simulink model "SF051A_SnsrOffsLrng"  (R2013b)
settings: Solver=FixedStepDiscrete  SolverMode=SingleTasking  StartTime=0.0  StopTime=1  FixedStep=0.002  RelTol=1e-3
values from neighbouring files (symbols this model uses):
  ARCHGLBPRM_10MILLISEC_SEC_F32 = DataDict.Constant    [SF051A_SnsrOffsLrng_DataDict.m]
  ARCHGLBPRM_2MILLISEC_SEC_F32 = DataDict.Constant    [SF051A_SnsrOffsLrng_DataDict.m]
  ARCHGLBPRM_2PI_ULS_F32 = DataDict.Constant    [SF051A_SnsrOffsLrng_DataDict.m]
  ARCHGLBPRM_FLOATZEROTHD_ULS_F32 = DataDict.Constant    [SF051A_SnsrOffsLrng_DataDict.m]
  ARCHGLBPRM_PIOVER180_ULS_F32 = DataDict.Constant    [SF051A_SnsrOffsLrng_DataDict.m]
  CNV100MICROSECTOSEC_SECPERCNT_F32 = DataDict.Constant    [SF051A_SnsrOffsLrng_DataDict.m]
  COVRAMTRXNIT_ULS_F32 = DataDict.Constant    [SF051A_SnsrOffsLrng_DataDict.m]
  HWAGHILIM_HWDEG_F32 = DataDict.Constant    [SF051A_SnsrOffsLrng_DataDict.m]
  HWAUTHYTHD_ULS_F32 = DataDict.Constant    [SF051A_SnsrOffsLrng_DataDict.m]
  HWTQLRNGSTSLRND_CNT_U08 = DataDict.Constant    [SF051A_SnsrOffsLrng_DataDict.m]
  HWTQLRNGSTSNEGOFFS_CNT_U08 = DataDict.Constant    [SF051A_SnsrOffsLrng_DataDict.m]
  HWTQLRNGSTSNOTLRND_CNT_U08 = DataDict.Constant    [SF051A_SnsrOffsLrng_DataDict.m]
  HWTQLRNGSTSPOSOFFS_CNT_U08 = DataDict.Constant    [SF051A_SnsrOffsLrng_DataDict.m]
  HWTQLRNGSTSZEROOFFS_CNT_U08 = DataDict.Constant    [SF051A_SnsrOffsLrng_DataDict.m]
  IDYMTRX_ULS_F32 = DataDict.Constant    [SF051A_SnsrOffsLrng_DataDict.m]
  IVS10MS_ULSPERSEC_F32 = DataDict.Constant    [SF051A_SnsrOffsLrng_DataDict.m]
  LRNGFILTICON_ULS_F32 = DataDict.Constant    [SF051A_SnsrOffsLrng_DataDict.m]
  ONE_ULS_F32 = DataDict.Constant    [SF051A_SnsrOffsLrng_DataDict.m]
  SnsrOffsLrnd = DataDict.NVM    [SF051A_SnsrOffsLrng_DataDict.m]
  SnsrOffsLrngFctEna = DataDict.Calibration    [SF051A_SnsrOffsLrng_DataDict.m]
  SnsrOffsLrngHwAgLrngDrvgDstThd = DataDict.Calibration    [SF051A_SnsrOffsLrng_DataDict.m]
  SnsrOffsLrngHwAgLrngEna = DataDict.Calibration    [SF051A_SnsrOffsLrng_DataDict.m]
  SnsrOffsLrngHwAgLrngHwVelThd = DataDict.Calibration    [SF051A_SnsrOffsLrng_DataDict.m]
  SnsrOffsLrngHwAgLrngSysTqThd = DataDict.Calibration    [SF051A_SnsrOffsLrng_DataDict.m]
  SnsrOffsLrngHwAgLrngSysTqThdMed = DataDict.Calibration    [SF051A_SnsrOffsLrng_DataDict.m]
  SnsrOffsLrngHwAgLrngSysTqThdTrustd = DataDict.Calibration    [SF051A_SnsrOffsLrng_DataDict.m]
  SnsrOffsLrngHwAgLrngSysTqThdWide = DataDict.Calibration    [SF051A_SnsrOffsLrng_DataDict.m]
  SnsrOffsLrngHwAgLrngTi = DataDict.Calibration    [SF051A_SnsrOffsLrng_DataDict.m]
  SnsrOffsLrngHwAgLrngVehSpdThd = DataDict.Calibration    [SF051A_SnsrOffsLrng_DataDict.m]
  SnsrOffsLrngHwAgLrngYawOffsDbnd = DataDict.Calibration    [SF051A_SnsrOffsLrng_DataDict.m]
  SnsrOffsLrngHwAgLrngYawRateThd = DataDict.Calibration    [SF051A_SnsrOffsLrng_DataDict.m]
  SnsrOffsLrngHwAgOffsLim = DataDict.Calibration    [SF051A_SnsrOffsLrng_DataDict.m]
  SnsrOffsLrngHwTqLrngEna = DataDict.Calibration    [SF051A_SnsrOffsLrng_DataDict.m]
  SnsrOffsLrngHwTqLrngEnaTiThd = DataDict.Calibration    [SF051A_SnsrOffsLrng_DataDict.m]
  SnsrOffsLrngHwTqLrngHwAgDbnd = DataDict.Calibration    [SF051A_SnsrOffsLrng_DataDict.m]
  SnsrOffsLrngHwTqLrngHwAgThd = DataDict.Calibration    [SF051A_SnsrOffsLrng_DataDict.m]
  SnsrOffsLrngHwTqLrngHwTqThd = DataDict.Calibration    [SF051A_SnsrOffsLrng_DataDict.m]
  SnsrOffsLrngHwTqLrngHwTqZeroOffsThd = DataDict.Calibration    [SF051A_SnsrOffsLrng_DataDict.m]
  SnsrOffsLrngHwTqLrngHwVelThd = DataDict.Calibration    [SF051A_SnsrOffsLrng_DataDict.m]
  SnsrOffsLrngHwTqLrngMeasTi = DataDict.Calibration    [SF051A_SnsrOffsLrng_DataDict.m]
  SnsrOffsLrngHwTqLrngMeasTiScar = DataDict.Calibration    [SF051A_SnsrOffsLrng_DataDict.m]
  SnsrOffsLrngHwTqLrngSampleImbThd1 = DataDict.Calibration    [SF051A_SnsrOffsLrng_DataDict.m]
  SnsrOffsLrngHwTqLrngSampleImbThd2 = DataDict.Calibration    [SF051A_SnsrOffsLrng_DataDict.m]
  SnsrOffsLrngHwTqLrngSampleThd1 = DataDict.Calibration    [SF051A_SnsrOffsLrng_DataDict.m]
  SnsrOffsLrngHwTqLrngSampleThd2 = DataDict.Calibration    [SF051A_SnsrOffsLrng_DataDict.m]
  SnsrOffsLrngHwTqLrngTiWghtCoeff = DataDict.Calibration    [SF051A_SnsrOffsLrng_DataDict.m]
  SnsrOffsLrngHwTqLrngVehSpdThd = DataDict.Calibration    [SF051A_SnsrOffsLrng_DataDict.m]
  SnsrOffsLrngHwTqOffsLim = DataDict.Calibration    [SF051A_SnsrOffsLrng_DataDict.m]
  SnsrOffsLrngSampleCntForHwTqLrngRst = DataDict.Calibration    [SF051A_SnsrOffsLrng_DataDict.m]
  SnsrOffsLrngTqInpDetnPwrEstimnThd = DataDict.Calibration    [SF051A_SnsrOffsLrng_DataDict.m]
  SnsrOffsLrngTqInpDetnSinGenrAmp = DataDict.Calibration    [SF051A_SnsrOffsLrng_DataDict.m]
  SnsrOffsLrngTqInpDetnSinGenrFrq = DataDict.Calibration    [SF051A_SnsrOffsLrng_DataDict.m]
  SnsrOffsLrngTqInpDetnStg1FilGain = DataDict.Calibration    [SF051A_SnsrOffsLrng_DataDict.m]
  SnsrOffsLrngTqInpDetnStg1WinSize = DataDict.Calibration    [SF051A_SnsrOffsLrng_DataDict.m]
  SnsrOffsLrngTqInpDetnStg2FilGainCen = DataDict.Calibration    [SF051A_SnsrOffsLrng_DataDict.m]
  SnsrOffsLrngTqInpDetnStg2FilGainDwn = DataDict.Calibration    [SF051A_SnsrOffsLrng_DataDict.m]
  SnsrOffsLrngTqInpDetnStg2FilGainUp = DataDict.Calibration    [SF051A_SnsrOffsLrng_DataDict.m]
  SnsrOffsLrngTqInpDetnStg2WinSize = DataDict.Calibration    [SF051A_SnsrOffsLrng_DataDict.m]
  SnsrOffsLrngYawLrngEna = DataDict.Calibration    [SF051A_SnsrOffsLrng_DataDict.m]
  SnsrOffsLrngYawLrngHwAgThd = DataDict.Calibration    [SF051A_SnsrOffsLrng_DataDict.m]
  SnsrOffsLrngYawLrngTi = DataDict.Calibration    [SF051A_SnsrOffsLrng_DataDict.m]
  SnsrOffsLrngYawLrngYawAThd = DataDict.Calibration    [SF051A_SnsrOffsLrng_DataDict.m]
  SnsrOffsLrngYawOffsFrshTiThd = DataDict.Calibration    [SF051A_SnsrOffsLrng_DataDict.m]
  SnsrOffsLrngYawRateOffsLim = DataDict.Calibration    [SF051A_SnsrOffsLrng_DataDict.m]
  SPDCNVN_MTRPERSECPERKPH_F32 = DataDict.Constant    [SF051A_SnsrOffsLrng_DataDict.m]
  SysGlbPrmSysTqRat = DataDict.ImprtdCal    [SF051A_SnsrOffsLrng_DataDict.m]
  TISTEP10MS_MINS_F32 = DataDict.Constant    [SF051A_SnsrOffsLrng_DataDict.m]
  TQINPDETNLOGGAIN_ULS_F32 = DataDict.Constant    [SF051A_SnsrOffsLrng_DataDict.m]
  YAWELPDTIHILIM_MINS_F32 = DataDict.Constant    [SF051A_SnsrOffsLrng_DataDict.m]
  YAWRATENOISE_VEHDEGPERSEC_F32 = DataDict.Constant    [SF051A_SnsrOffsLrng_DataDict.m]
  ZERO_ULS_F32 = DataDict.Constant    [SF051A_SnsrOffsLrng_DataDict.m]
  ZEROVECT_ULS_F32 = DataDict.Constant    [SF051A_SnsrOffsLrng_DataDict.m]
undefined symbols (not defined in the file or in its folder): NvmGetErrSts1
libraries: Fil x34, NxtrLim x20, FixdToFloat x17, FloatToFixd x16, simulink x12, NxtrAbslt x12, NxtrNvM x8, NxtrMath x3
(part 8 of 12)

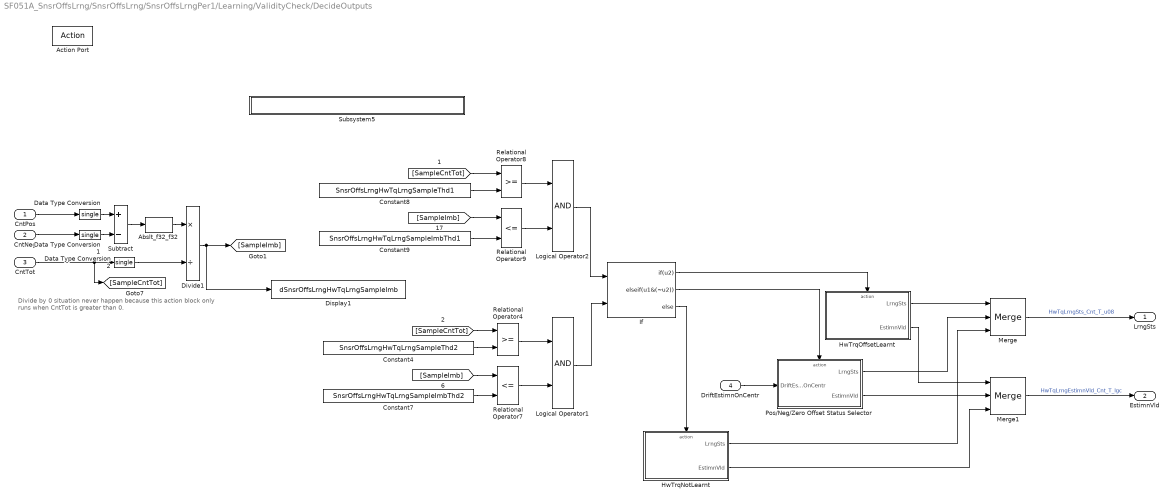
== system SF051A_SnsrOffsLrng/SnsrOffsLrng/SnsrOffsLrngPer1/Learning/ValidityCheck/DecideOutputs ==
  note: Divide by 0 situation never happen because this
      | action block only runs when CntTot is greater than 0.
  CntPos : Inport
  CntNeg : Inport  Port=2
  CntTot : Inport  Port=3
  DriftEstimnOnCentr : Inport  Port=4
  Action Port : ActionPort  ActionType=then
  Abslt_f32_f32 : NxtrAbslt/Abslt_f32_f32  SFunctionSpec=single y1 = Abslt_f32_f32(single u1)
      settings: AttributesFormatString=%<Name>
  Constant4 : Constant  RequirementInfo="{'linktype_rmi_doors' '0000babd (/E-STEER Core/SubSystem Specifications/Application Functions/SF051A Sensor Offset Learning)' '#SF051A_191' 'true' 'REQ:  SF051A_191' '' } %GIDa_69e41f1c_0c44_40e9_b72f_03bb47ca0505"  Value=SnsrOffsLrngHwTqLrngSampleThd2
  Constant7 : Constant  RequirementInfo="{'linktype_rmi_doors' '0000babd (/E-STEER Core/SubSystem Specifications/Application Functions/SF051A Sensor Offset Learning)' '#SF051A_191' 'true' 'REQ:  SF051A_191' '' } %GIDa_92758992_3392_4f8d_bbc2_47c47a841263"  Value=SnsrOffsLrngHwTqLrngSampleImbThd2
  Constant8 : Constant  RequirementInfo="{'linktype_rmi_doors' '0000babd (/E-STEER Core/SubSystem Specifications/Application Functions/SF051A Sensor Offset Learning)' '#SF051A_186' 'true' 'REQ: SF051A_186' '' ; 'linktype_rmi_doors' '0000babd (/E-STEER Core/SubSystem Specifications/Application Functions/SF051A Sensor Offset Learning)' '#SF051A_195' 'true' 'REQ:  SF051A_195' '' ; 'linktype_rmi_doors' '0000babd (/E-STEER Core/SubSystem Specifications/Application Functions/SF051A Sensor Offset Learning)' '#SF051A_194' 'true' 'REQ:  SF051A_194' '' } %GIDa_ce699618_5d0a_4879_9841_5152f833be51"  Value=SnsrOffsLrngHwTqLrngSampleThd1
  Constant9 : Constant  RequirementInfo="{'linktype_rmi_doors' '0000babd (/E-STEER Core/SubSystem Specifications/Application Functions/SF051A Sensor Offset Learning)' '#SF051A_186' 'true' 'REQ: SF051A_186' '' ; 'linktype_rmi_doors' '0000babd (/E-STEER Core/SubSystem Specifications/Application Functions/SF051A Sensor Offset Learning)' '#SF051A_195' 'true' 'REQ:  SF051A_195' '' ; 'linktype_rmi_doors' '0000babd (/E-STEER Core/SubSystem Specifications/Application Functions/SF051A Sensor Offset Learning)' '#SF051A_194' 'true' 'REQ:  SF051A_194' '' } %GIDa_77d3a507_06ae_4bbf_9b68_48e8353a45e0"  Value=SnsrOffsLrngHwTqLrngSampleImbThd1
  Data Type Conversion : DataTypeConversion  OutDataTypeStr=single
  Data Type Conversion1 : DataTypeConversion  OutDataTypeStr=single
  Data Type Conversion2 : DataTypeConversion  OutDataTypeStr=single
  Display1 : DataStoreWrite  DataStoreName=dSnsrOffsLrngHwTqLrngSampleImb
  Divide1 : Product  Inputs=*/
  HwTrqNotLearnt : Subsystem  RequirementInfo="{'linktype_rmi_doors' '0000babd (/E-STEER Core/SubSystem Specifications/Application Functions/SF051A Sensor Offset Learning)' '#SF051A_188' 'true' 'REQ:  SF051A_188' '' } %GIDa_0852b3e3_8f60_4c1b_a1ce_1713cda0b42d"  TreatAsAtomicUnit=on
  HwTrqOffsetLearnt : Subsystem  RequirementInfo="{'linktype_rmi_doors' '0000babd (/E-STEER Core/SubSystem Specifications/Application Functions/SF051A Sensor Offset Learning)' '#SF051A_191' 'true' 'REQ:  SF051A_191' '' ; 'linktype_rmi_doors' '0000babd (/E-STEER Core/SubSystem Specifications/Application Functions/SF051A Sensor Offset Learning)' '#SF051A_187' 'true' 'REQ:  SF051A_187' '' } %GIDa_a502fd14_57b6_42c3_a417_d587305743af"  TreatAsAtomicUnit=on
  If : If  RequirementInfo="{'linktype_rmi_doors' '0000babd (/E-STEER Core/SubSystem Specifications/Application Functions/SF051A Sensor Offset Learning)' '#SF051A_191' 'true' 'REQ: SF051A_191' '' ; 'linktype_rmi_doors' '0000babd (/E-STEER Core/SubSystem Specifications/Application Functions/SF051A Sensor Offset Learning)' '#SF051A_188' 'true' 'REQ:  SF051A_188' '' ; 'linktype_rmi_doors' '0000babd (/E-STEER Core/SubSystem Specifications/Application Functions/SF051A Sensor Offset Learning)' '#SF051A_187' 'true' 'REQ:  SF051A_187' '' ; 'linktype_rmi_doors' '0000babd (/E-STEER Core/SubSystem Specifications/Application Functions/SF051A Sensor Offset Learning)' '#SF051A_186' 'true' 'REQ:  SF051A_186' '' ; 'linktype_rmi_doors' '0000babd (/E-STEER Core/SubSystem Specifications/Application Functions/SF051A Sensor Offset Learning)' '#SF051A_195' 'true' 'REQ:  SF051A_195' '' ; 'linktype_rmi_doors' '0000babd (/E-STEER Core/SubSystem Specifications/Application Functions/SF051A Sensor Offset Learning)' '#SF051A_194' 'true' 'REQ:  SF051A_194' '' } %GIDa_3b80c21c_9329_459d_81b8_15c83f98be44"  NumInputs=2  IfExpression=u2  ElseIfExpressions=u1&(~u2)
  Logical Operator1 : Logic  RequirementInfo="{'linktype_rmi_doors' '0000babd (/E-STEER Core/SubSystem Specifications/Application Functions/SF051A Sensor Offset Learning)' '#SF051A_191' 'true' 'REQ:  SF051A_191' '' } %GIDa_0d8d9f4f_132b_432e_bde6_871d76097d27"  AllPortsSameDT=off  OutDataTypeStr=boolean
  Logical Operator2 : Logic  RequirementInfo="{'linktype_rmi_doors' '0000babd (/E-STEER Core/SubSystem Specifications/Application Functions/SF051A Sensor Offset Learning)' '#SF051A_186' 'true' 'REQ: SF051A_186' '' ; 'linktype_rmi_doors' '0000babd (/E-STEER Core/SubSystem Specifications/Application Functions/SF051A Sensor Offset Learning)' '#SF051A_195' 'true' 'REQ:  SF051A_195' '' ; 'linktype_rmi_doors' '0000babd (/E-STEER Core/SubSystem Specifications/Application Functions/SF051A Sensor Offset Learning)' '#SF051A_194' 'true' 'REQ:  SF051A_194' '' } %GIDa_51f40efb_db01_49b1_90e1_88342bdb2bcc"  AllPortsSameDT=off  OutDataTypeStr=boolean
  Merge : Merge  Inputs=3
  Merge1 : Merge  Inputs=3
  Pos/Neg/Zero Offset Status Selector : Subsystem  TreatAsAtomicUnit=on
  Relational Operator4 : RelationalOperator  RequirementInfo="{'linktype_rmi_doors' '0000babd (/E-STEER Core/SubSystem Specifications/Application Functions/SF051A Sensor Offset Learning)' '#SF051A_191' 'true' 'REQ:  SF051A_191' '' } %GIDa_e4ce5424_fe6e_4165_9ce9_8a105b03caf7"  OutDataTypeStr=boolean
  Relational Operator7 : RelationalOperator  RequirementInfo="{'linktype_rmi_doors' '0000babd (/E-STEER Core/SubSystem Specifications/Application Functions/SF051A Sensor Offset Learning)' '#SF051A_191' 'true' 'REQ:  SF051A_191' '' } %GIDa_9020cee8_144c_4ac3_9e5a_358b6b128393"  Operator=<=  OutDataTypeStr=boolean
  Relational Operator8 : RelationalOperator  RequirementInfo="{'linktype_rmi_doors' '0000babd (/E-STEER Core/SubSystem Specifications/Application Functions/SF051A Sensor Offset Learning)' '#SF051A_186' 'true' 'REQ: SF051A_186' '' ; 'linktype_rmi_doors' '0000babd (/E-STEER Core/SubSystem Specifications/Application Functions/SF051A Sensor Offset Learning)' '#SF051A_195' 'true' 'REQ:  SF051A_195' '' ; 'linktype_rmi_doors' '0000babd (/E-STEER Core/SubSystem Specifications/Application Functions/SF051A Sensor Offset Learning)' '#SF051A_194' 'true' 'REQ:  SF051A_194' '' } %GIDa_6066e143_82e9_483a_abba_1d193ece918f"  OutDataTypeStr=boolean
  Relational Operator9 : RelationalOperator  RequirementInfo="{'linktype_rmi_doors' '0000babd (/E-STEER Core/SubSystem Specifications/Application Functions/SF051A Sensor Offset Learning)' '#SF051A_186' 'true' 'REQ: SF051A_186' '' ; 'linktype_rmi_doors' '0000babd (/E-STEER Core/SubSystem Specifications/Application Functions/SF051A Sensor Offset Learning)' '#SF051A_195' 'true' 'REQ:  SF051A_195' '' ; 'linktype_rmi_doors' '0000babd (/E-STEER Core/SubSystem Specifications/Application Functions/SF051A Sensor Offset Learning)' '#SF051A_194' 'true' 'REQ:  SF051A_194' '' } %GIDa_e5c9dca8_a081_4dd4_a606_b25af821b798"  Operator=<=  OutDataTypeStr=boolean
  Subsystem5 : Subsystem  Description=|  mask(Copyright Information){none=on}
      | Copyright info block.                                               
      |                                                                     
      | Place copyright information at the top of every subsystem in design.
      mask prompts: none "No parameters"
      mask help: Place copyright information at the top of every subsystem in design.
      mask Display:
      | NxtrConf = 'Nexteer Confidential';
      | 
      | sys = bdroot; %handle for the current model ("system")
      | first = get_param(sys,'Created');
      | first = first(end-3:end);  %year is last four digits
      | 
      | last = get_param(sys,'LastModifiedDate');
      | if isempty(last)
      |     last = datestr(now,'yyyy');
      | else
      |     last = last(end-3:end);
      | end
      | 
      | if strcmp(first,last)
      |     fprintf('%s -- Copyright %s Nexteer',NxtrConf,first)
      | else
      |     fprintf('%s -- %s%s- %s Nexteer',NxtrConf,char(169),first,last)
      | end
  Subtract : Sum  Inputs=+-
  LrngSts : Outport
  EstimnVld : Outport  Port=2
  wires:
  Constant4/1 -> Relational Operator4/2
  [SampleCntTot] -> Relational Operator4/1
  Constant7/1 -> Relational Operator7/2
  Relational Operator7/1 -> Logical Operator1/2
  Logical Operator1/1 -> If/2
  Constant8/1 -> Relational Operator8/2
  [SampleCntTot] -> Relational Operator8/1
  Relational Operator8/1 -> Logical Operator2/1
  Subtract/1 -> Abslt_f32_f32/1
  Abslt_f32_f32/1 -> Divide1/1
  CntNeg/1 -> Data Type Conversion1/1
  CntPos/1 -> Data Type Conversion/1
  [SampleImb] -> Relational Operator7/1
  Constant9/1 -> Relational Operator9/2
  [SampleImb] -> Relational Operator9/1
  Relational Operator9/1 -> Logical Operator2/2
  Relational Operator4/1 -> Logical Operator1/1
  Logical Operator2/1 -> If/1
  If/1 -> HwTrqOffsetLearnt/Action
  DriftEstimnOnCentr/1 -> Pos/Neg/Zero Offset Status Selector/1(DriftEstimnOnCentr)
  If/2 -> Pos/Neg/Zero Offset Status Selector/Action
  Merge/1 -> LrngSts/1  "HwTqLrngSts_Cnt_T_u08"
  Merge1/1 -> EstimnVld/1  "HwTqLrngEstimnVld_Cnt_T_lgc"
  HwTrqNotLearnt/1(LrngSts) -> Merge/3
  HwTrqNotLearnt/2(EstimnVld) -> Merge1/3
  Pos/Neg/Zero Offset Status Selector/2(EstimnVld) -> Merge1/2
  Pos/Neg/Zero Offset Status Selector/1(LrngSts) -> Merge/2
  HwTrqOffsetLearnt/1(LrngSts) -> Merge/1
  If/3 -> HwTrqNotLearnt/Action
  HwTrqOffsetLearnt/2(EstimnVld) -> Merge1/1
  Data Type Conversion/1 -> Subtract/1
  Data Type Conversion1/1 -> Subtract/2
  Data Type Conversion2/1 -> Divide1/2
  Divide1/1 -> Display1/1, [SampleImb]
  CntTot/1 -> [SampleCntTot], Data Type Conversion2/1

== system SF051A_SnsrOffsLrng/SnsrOffsLrng/SnsrOffsLrngPer1/Learning/ValidityCheck/HwTrqNotLearnt ==
  note: TOCStatus
      | 0 = HwTrq NotLearnt
      | 1 = Positive HwTrq Offset
      | 2 = Negative HwTrqOffset
      | 3 = Zero HwTrq Offset
      | 4 = HwTrq Offset Learnt
  Action Port : ActionPort  ActionType=else
  Constant1 : Constant  Value=false  OutDataTypeStr=boolean
      settings: AttributesFormatString=%<OutDataTypeStr>
  Constant3 : Constant  Value=HWTQLRNGSTSNOTLRND_CNT_U08  OutDataTypeStr=uint8
  Subsystem5 : Subsystem  Description=|  mask(Copyright Information){none=on}
      | Copyright info block.                                               
      |                                                                     
      | Place copyright information at the top of every subsystem in design.
      mask prompts: none "No parameters"
      mask help: Place copyright information at the top of every subsystem in design.
      mask Display:
      | NxtrConf = 'Nexteer Confidential';
      | 
      | sys = bdroot; %handle for the current model ("system")
      | first = get_param(sys,'Created');
      | first = first(end-3:end);  %year is last four digits
      | 
      | last = get_param(sys,'LastModifiedDate');
      | if isempty(last)
      |     last = datestr(now,'yyyy');
      | else
      |     last = last(end-3:end);
      | end
      | 
      | if strcmp(first,last)
      |     fprintf('%s -- Copyright %s Nexteer',NxtrConf,first)
      | else
      |     fprintf('%s -- %s%s- %s Nexteer',NxtrConf,char(169),first,last)
      | end
  LrngSts : Outport
  EstimnVld : Outport  Port=2
  wires:
  Constant3/1 -> LrngSts/1
  Constant1/1 -> EstimnVld/1

== system SF051A_SnsrOffsLrng/SnsrOffsLrng/SnsrOffsLrngPer1/Learning/ValidityCheck/Subsystem5 ==

== system SF051A_SnsrOffsLrng/SnsrOffsLrng/SnsrOffsLrngPer1/Measurements_Grabber/False/Subsystem5 ==

== system SF051A_SnsrOffsLrng/SnsrOffsLrng/SnsrOffsLrngPer1/Measurements_Grabber/GetTiSpan100MicroSec32bit/CopyRight2 ==

== system SF051A_SnsrOffsLrng/SnsrOffsLrng/SnsrOffsLrngPer1/Measurements_Grabber/GetTiSpan100MicroSec32bit/No wrapping ==
  new : Inport
  ref : Inport  Port=2
  Action Port : ActionPort  ActionType=then
  CopyRight2 : Subsystem  Description=|  mask(Copyright Information){none=on}
      | Copyright info block.                                               
      |                                                                     
      | Place copyright information at the top of every subsystem in design.
      mask prompts: none "No parameters"
      mask help: Place copyright information at the top of every subsystem in design.
      mask Display:
      | NxtrConf = 'Nexteer Confidential';
      | 
      | sys = bdroot; %handle for the current model ("system")
      | first = get_param(sys,'Created');
      | if(isempty(first))
      |     first = datestr(now,'yyyy');
      | else
      |     first = first(end-3:end);  %year is last four digits
      | end
      | 
      | last = get_param(sys,'LastModifiedDate');
      | if isempty(last)
      |     last = datestr(now,'yyyy');
      | else
      |     last = last(end-3:end);
      | end
      | 
      | if strcmp(first,last)
      |     fprintf('%s -- Copyright %s Nexteer',NxtrConf,first)
      | else
      |     fprintf('%s -- %s%s- %s Nexteer',NxtrConf,char(169),first,last)
      | end
  Subtract1 : Sum  Inputs=+-
  Out1 : Outport
  wires:
  ref/1 -> Subtract1/2
  new/1 -> Subtract1/1
  Subtract1/1 -> Out1/1

== system SF051A_SnsrOffsLrng/SnsrOffsLrng/SnsrOffsLrngPer1/Measurements_Grabber/GetTiSpan100MicroSec32bit/Wrapping ==
  new : Inport
  ref : Inport  Port=2
  Action Port : ActionPort  ActionType=else
  CopyRight2 : Subsystem  Description=|  mask(Copyright Information){none=on}
      | Copyright info block.                                               
      |                                                                     
      | Place copyright information at the top of every subsystem in design.
      mask prompts: none "No parameters"
      mask help: Place copyright information at the top of every subsystem in design.
      mask Display:
      | NxtrConf = 'Nexteer Confidential';
      | 
      | sys = bdroot; %handle for the current model ("system")
      | first = get_param(sys,'Created');
      | if(isempty(first))
      |     first = datestr(now,'yyyy');
      | else
      |     first = first(end-3:end);  %year is last four digits
      | end
      | 
      | last = get_param(sys,'LastModifiedDate');
      | if isempty(last)
      |     last = datestr(now,'yyyy');
      | else
      |     last = last(end-3:end);
      | end
      | 
      | if strcmp(first,last)
      |     fprintf('%s -- Copyright %s Nexteer',NxtrConf,first)
      | else
      |     fprintf('%s -- %s%s- %s Nexteer',NxtrConf,char(169),first,last)
      | end
  Max Counts : Constant  Value=2^32-1  OutDataTypeStr=uint32
  Subtract1 : Sum  Inputs=+-+
  Out1 : Outport
  wires:
  new/1 -> Subtract1/3
  ref/1 -> Subtract1/2
  Max Counts/1 -> Subtract1/1
  Subtract1/1 -> Out1/1

== system SF051A_SnsrOffsLrng/SnsrOffsLrng/SnsrOffsLrngPer1/Measurements_Grabber/True_UpdateNVMRam/GetRefTmr100MicroSec32bit ==
  note: 1 count = 100 uSec
  note: seconds
  note: microseconds
  note: counts
  note: Wrap-to-zero
  note: GetRefTmr100MicroSec32bit
  note: Created Aug 18, 2015
      | Modified Oct 21, 2015
      | Modified Oct 30, 2015
      | Kevin Derry
  CopyRight2 : Subsystem  Description=|  mask(Copyright Information){none=on}
      | Copyright info block.                                               
      |                                                                     
      | Place copyright information at the top of every subsystem in design.
      mask prompts: none "No parameters"
      mask help: Place copyright information at the top of every subsystem in design.
      mask Display:
      | NxtrConf = 'Nexteer Confidential';
      | 
      | sys = bdroot; %handle for the current model ("system")
      | first = get_param(sys,'Created');
      | if(isempty(first))
      |     first = datestr(now,'yyyy');
      | else
      |     first = first(end-3:end);  %year is last four digits
      | end
      | 
      | last = get_param(sys,'LastModifiedDate');
      | if isempty(last)
      |     last = datestr(now,'yyyy');
      | else
      |     last = last(end-3:end);
      | end
      | 
      | if strcmp(first,last)
      |     fprintf('%s -- Copyright %s Nexteer',NxtrConf,first)
      | else
      |     fprintf('%s -- %s%s- %s Nexteer',NxtrConf,char(169),first,last)
      | end
  Count per uSec : Constant  Value=0.01
  Data Store Read1 : DataStoreRead  DataStoreName=SimnTi
  Data Type Conversion1 : DataTypeConversion  OutDataTypeStr=uint32
  Divide1 : Product  Inputs=**
  Divide2 : Product  Inputs=*/
  Max Counts : Constant  Value=2^32-1
  Product1 : Product
  Product2 : Product
  Rounding : Rounding
  Subtract1 : Sum  Inputs=+-
  uSec per Sec : Constant  Value=1000000
  RefTmr : Outport
  wires:
  Product2/1 -> Subtract1/2
  Subtract1/1 -> Data Type Conversion1/1
  Rounding/1 -> Product2/1
  Divide2/1 -> Rounding/1
  Max Counts/1 -> Divide2/2, Product2/2
  Divide1/1 -> Divide2/1, Subtract1/1
  Product1/1 -> Divide1/1
  Count per uSec/1 -> Divide1/2
  uSec per Sec/1 -> Product1/2
  Data Type Conversion1/1 -> RefTmr/1
  Data Store Read1/1 -> Product1/1

== system SF051A_SnsrOffsLrng/SnsrOffsLrng/SnsrOffsLrngPer1/Measurements_Grabber/True_UpdateNVMRam/Subsystem5 ==

== system SF051A_SnsrOffsLrng/SnsrOffsLrng/SnsrOffsLrngPer1/Zero_GrabberTimer/GetRefTmr100MicroSec32bit/CopyRight2 ==

== system SF051A_SnsrOffsLrng/SnsrOffsLrng/SnsrOffsLrngPer2/Enable_Function/Condition Signals/Subsystem5 ==

== system SF051A_SnsrOffsLrng/SnsrOffsLrng/SnsrOffsLrngPer2/Enable_Function/POC/Do nothing ==
  Action Port : ActionPort  ActionType=else
  Subsystem5 : Subsystem  Description=|  mask(Copyright Information){none=on}
      | Copyright info block.                                               
      |                                                                     
      | Place copyright information at the top of every subsystem in design.
      mask prompts: none "No parameters"
      mask help: Place copyright information at the top of every subsystem in design.
      mask Display:
      | NxtrConf = 'Nexteer Confidential';
      | 
      | sys = bdroot; %handle for the current model ("system")
      | first = get_param(sys,'Created');
      | first = first(end-3:end);  %year is last four digits
      | 
      | last = get_param(sys,'LastModifiedDate');
      | if isempty(last)
      |     last = datestr(now,'yyyy');
      | else
      |     last = last(end-3:end);
      | end
      | 
      | if strcmp(first,last)
      |     fprintf('%s -- Copyright %s Nexteer',NxtrConf,first)
      | else
      |     fprintf('%s -- %s%s- %s Nexteer',NxtrConf,char(169),first,last)
      | end

== system SF051A_SnsrOffsLrng/SnsrOffsLrng/SnsrOffsLrngPer2/Enable_Function/POC/Do nothing1 ==
  Action Port : ActionPort  ActionType=else
  Subsystem5 : Subsystem  Description=|  mask(Copyright Information){none=on}
      | Copyright info block.                                               
      |                                                                     
      | Place copyright information at the top of every subsystem in design.
      mask prompts: none "No parameters"
      mask help: Place copyright information at the top of every subsystem in design.
      mask Display:
      | NxtrConf = 'Nexteer Confidential';
      | 
      | sys = bdroot; %handle for the current model ("system")
      | first = get_param(sys,'Created');
      | first = first(end-3:end);  %year is last four digits
      | 
      | last = get_param(sys,'LastModifiedDate');
      | if isempty(last)
      |     last = datestr(now,'yyyy');
      | else
      |     last = last(end-3:end);
      | end
      | 
      | if strcmp(first,last)
      |     fprintf('%s -- Copyright %s Nexteer',NxtrConf,first)
      | else
      |     fprintf('%s -- %s%s- %s Nexteer',NxtrConf,char(169),first,last)
      | end

== system SF051A_SnsrOffsLrng/SnsrOffsLrng/SnsrOffsLrngPer2/Enable_Function/POC/Learn ==
  note: When the BiasEstimator block is disabled after being enabled,
      | the latest states of the learning filters and timer must be saved and recovered
      | next time that the BiasEstimator block is enabled.
      | The state of the learning filters and timer shall be saved also between
      | ignition cycles.
  HwAgFild : Inport
  SysTrqFild : Inport  Port=2
  HwTqLrngSts : Inport  Port=3
  Action Port : ActionPort  ActionType=then
  BiasEstimation_ValidityCheck : Subsystem
  LPFs : Subsystem  RequirementInfo="{'linktype_rmi_doors' '0000babd (/E-STEER Core/SubSystem Specifications/Application Functions/SF051A Sensor Offset Learning)' '#SF051A_123' 'true' 'REQ:  SF051A_123' '' } %GIDa_6c88d437_3f63_4750_9609_e2b4b1ce4a68"
  Subsystem5 : Subsystem  Description=|  mask(Copyright Information){none=on}
      | Copyright info block.                                               
      |                                                                     
      | Place copyright information at the top of every subsystem in design.
      mask prompts: none "No parameters"
      mask help: Place copyright information at the top of every subsystem in design.
      mask Display:
      | NxtrConf = 'Nexteer Confidential';
      | 
      | sys = bdroot; %handle for the current model ("system")
      | first = get_param(sys,'Created');
      | first = first(end-3:end);  %year is last four digits
      | 
      | last = get_param(sys,'LastModifiedDate');
      | if isempty(last)
      |     last = datestr(now,'yyyy');
      | else
      |     last = last(end-3:end);
      | end
      | 
      | if strcmp(first,last)
      |     fprintf('%s -- Copyright %s Nexteer',NxtrConf,first)
      | else
      |     fprintf('%s -- %s%s- %s Nexteer',NxtrConf,char(169),first,last)
      | end
  wires:
  HwAgFild/1 -> LPFs/1(HwAgFild)
  SysTrqFild/1 -> LPFs/2(SysTqFild)
  LPFs/3(SysTqAvrg) -> BiasEstimation_ValidityCheck/4(SysTqAvrg)
  LPFs/1(ElpsdTi) -> BiasEstimation_ValidityCheck/2(ElpsdTi)
  LPFs/2(HwPosBiasEstRaw) -> BiasEstimation_ValidityCheck/3(HwPosBiasEstRaw)
  HwTqLrngSts/1 -> BiasEstimation_ValidityCheck/1(HwTqLrngSts)

== system SF051A_SnsrOffsLrng/SnsrOffsLrng/SnsrOffsLrngPer2/Enable_Function/POC/Learning Conditions ==
  note: Learning is activated after a certain travelled distance
      |  with all the enablers being true.
  note: InputTrq prevents learning while driving straight
      | on a highly cambered road.
  note: HwVel enabler ensures that the learning is not enabled
      | during YawRate transitions or zero-crossing.
  note: VehSpd enabler ensures that the vehicle is over a determinate speed.
      | The higher the VehSpd, the more sensitive is the YawRate to HwPos
      | changes. This improves the driving straight detection based on YawRate.
  note: Main enabler (tighter Threshold) is the Yaw rate
      | signal. When equal to 0 DegpS, indicates that
      | the vehicle is driving straight.
  VehSpd : Inport  RequirementInfo="{'linktype_rmi_doors' '0000babd (/E-STEER Core/SubSystem Specifications/Application Functions/SF051A Sensor Offset Learning)' '#SF051A_125' 'true' 'REQ:  SF051A_125' '' } %GIDa_8f59ea37_a6d2_43e8_9752_10147a2ef345"
  HwVelFild : Inport  RequirementInfo="{'linktype_rmi_doors' '0000babd (/E-STEER Core/SubSystem Specifications/Application Functions/SF051A Sensor Offset Learning)' '#SF051A_125' 'true' 'REQ:  SF051A_125' '' } %GIDa_b4c3f45d_537f_4ddb_98c2_1cbec19599c7"  Port=2
  YawRateCorrd : Inport  RequirementInfo="{'linktype_rmi_doors' '0000babd (/E-STEER Core/SubSystem Specifications/Application Functions/SF051A Sensor Offset Learning)' '#SF051A_125' 'true' 'REQ:  SF051A_125' '' } %GIDa_f2d4e035_e9df_4867_bc0f_7342acf6aef2"  Port=3
  SysTqFild : Inport  RequirementInfo="{'linktype_rmi_doors' '0000babd (/E-STEER Core/SubSystem Specifications/Application Functions/SF051A Sensor Offset Learning)' '#SF051A_125' 'true' 'REQ:  SF051A_125' '' } %GIDa_89d517e6_3be2_4d40_b33c_782ff70a0841"  Port=4
  Abslt_f32_f1 : NxtrAbslt/Abslt_f32_f32  RequirementInfo="{'linktype_rmi_doors' '0000babd (/E-STEER Core/SubSystem Specifications/Application Functions/SF051A Sensor Offset Learning)' '#SF051A_125' 'true' 'REQ:  SF051A_125' '' } %GIDa_4a9ff294_23c2_4635_9f2d_79eead891ad6"  SFunctionSpec=single y1 = Abslt_f32_f32(single u1)
      settings: AttributesFormatString=%<Name>
  Abslt_f32_f2 : NxtrAbslt/Abslt_f32_f32  RequirementInfo="{'linktype_rmi_doors' '0000babd (/E-STEER Core/SubSystem Specifications/Application Functions/SF051A Sensor Offset Learning)' '#SF051A_125' 'true' 'REQ:  SF051A_125' '' } %GIDa_bfc6113a_71b3_4014_a79c_4dae946b5258"  SFunctionSpec=single y1 = Abslt_f32_f32(single u1)
      settings: AttributesFormatString=%<Name>
  Abslt_f32_f32 : NxtrAbslt/Abslt_f32_f32  RequirementInfo="{'linktype_rmi_doors' '0000babd (/E-STEER Core/SubSystem Specifications/Application Functions/SF051A Sensor Offset Learning)' '#SF051A_125' 'true' 'REQ:  SF051A_125' '' } %GIDa_d2113858_1e63_4f18_8ebd_0dfc37da8a17"  SFunctionSpec=single y1 = Abslt_f32_f32(single u1)
      settings: AttributesFormatString=%<Name>
  Calibration : Constant  RequirementInfo="{'linktype_rmi_doors' '0000babd (/E-STEER Core/SubSystem Specifications/Application Functions/SF051A Sensor Offset Learning)' '#SF051A_125' 'true' 'REQ:  SF051A_125' '' } %GIDa_a930c023_3647_4bfe_81cc_9ffe63be677e"  Value=SnsrOffsLrngHwAgLrngDrvgDstThd  OutDataTypeStr=single
  Constant : Constant  RequirementInfo="{'linktype_rmi_doors' '0000babd (/E-STEER Core/SubSystem Specifications/Application Functions/SF051A Sensor Offset Learning)' '#SF051A_125' 'true' 'REQ:  SF051A_125' '' } %GIDa_13ca1097_74d2_4314_ac4c_82655165c3ac"  Value=SnsrOffsLrngHwAgLrngHwVelThd
  Constant1 : Constant  RequirementInfo="{'linktype_rmi_doors' '0000babd (/E-STEER Core/SubSystem Specifications/Application Functions/SF051A Sensor Offset Learning)' '#SF051A_125' 'true' 'REQ:  SF051A_125' '' } %GIDa_f59d0f18_d8e0_4a0d_94a2_c992328d5f5a"  Value=SnsrOffsLrngHwAgLrngYawRateThd
  Constant2 : Constant  RequirementInfo="{'linktype_rmi_doors' '0000babd (/E-STEER Core/SubSystem Specifications/Application Functions/SF051A Sensor Offset Learning)' '#SF051A_125' 'true' 'REQ:  SF051A_125' '' } %GIDa_97889c00_0b86_483b_8ac6_8be83d1b4c7e"  Value=SnsrOffsLrngHwAgLrngSysTqThd
  Constant3 : Constant  RequirementInfo="{'linktype_rmi_doors' '0000babd (/E-STEER Core/SubSystem Specifications/Application Functions/SF051A Sensor Offset Learning)' '#SF051A_125' 'true' 'REQ:  SF051A_125' '' } %GIDa_891f1f78_3923_46ac_86af_9c596d3c2421"  Value=SnsrOffsLrngHwAgLrngVehSpdThd
  Data Store Write : DataStoreWrite  RequirementInfo="{'linktype_rmi_doors' '0000babd (/E-STEER Core/SubSystem Specifications/Application Functions/SF051A Sensor Offset Learning)' '#SF051A_125' 'true' 'REQ:  SF051A_125' '' } %GIDa_aa42ae09_446c_4add_b848_b1660a3a4485"  DataStoreName=HwAgLrngDrvgDstPrev
  Display : DataStoreWrite  DataStoreName=dSnsrOffsLrngHwAgLrngCdnVld
  DrivingStraight : Subsystem  RequirementInfo="{'linktype_rmi_doors' '0000babd (/E-STEER Core/SubSystem Specifications/Application Functions/SF051A Sensor Offset Learning)' '#SF051A_125' 'true' 'REQ:  SF051A_125' '' } %GIDa_cc37c45b_3205_4a2a_b2ac_e002ec0e3efb"  TreatAsAtomicUnit=on
  If : If  RequirementInfo="{'linktype_rmi_doors' '0000babd (/E-STEER Core/SubSystem Specifications/Application Functions/SF051A Sensor Offset Learning)' '#SF051A_125' 'true' 'REQ:  SF051A_125' '' } %GIDa_ada5f7e2_fce2_40ad_8932_f71606710b58"  NumInputs=4  IfExpression=u1&u2&u3&u4
  Merge : Merge  RequirementInfo="{'linktype_rmi_doors' '0000babd (/E-STEER Core/SubSystem Specifications/Application Functions/SF051A Sensor Offset Learning)' '#SF051A_125' 'true' 'REQ:  SF051A_125' '' } %GIDa_d84796a1_a26e_43c5_9d0e_55146953274b"
  NotDrivingStraight : Subsystem  RequirementInfo="{'linktype_rmi_doors' '0000babd (/E-STEER Core/SubSystem Specifications/Application Functions/SF051A Sensor Offset Learning)' '#SF051A_125' 'true' 'REQ:  SF051A_125' '' } %GIDa_0603d790_b5f5_4a89_b992_b3578dd6ccf7"  TreatAsAtomicUnit=on
  Relational Operator : RelationalOperator  RequirementInfo="{'linktype_rmi_doors' '0000babd (/E-STEER Core/SubSystem Specifications/Application Functions/SF051A Sensor Offset Learning)' '#SF051A_125' 'true' 'REQ:  SF051A_125' '' } %GIDa_f6c4f543_bc79_4284_beb0_7307c18ad0b4"  OutDataTypeStr=boolean
  Relational Operator1 : RelationalOperator  RequirementInfo="{'linktype_rmi_doors' '0000babd (/E-STEER Core/SubSystem Specifications/Application Functions/SF051A Sensor Offset Learning)' '#SF051A_125' 'true' 'REQ:  SF051A_125' '' } %GIDa_6196e2d7_d842_4412_b387_3769f28bfdab"  Operator=<=  OutDataTypeStr=boolean
  Relational Operator2 : RelationalOperator  RequirementInfo="{'linktype_rmi_doors' '0000babd (/E-STEER Core/SubSystem Specifications/Application Functions/SF051A Sensor Offset Learning)' '#SF051A_125' 'true' 'REQ:  SF051A_125' '' } %GIDa_70a60178_7c67_4179_9a47_94853d13d4d4"  Operator=<=  OutDataTypeStr=boolean
  Relational Operator3 : RelationalOperator  RequirementInfo="{'linktype_rmi_doors' '0000babd (/E-STEER Core/SubSystem Specifications/Application Functions/SF051A Sensor Offset Learning)' '#SF051A_125' 'true' 'REQ:  SF051A_125' '' } %GIDa_022c8ef0_d08f_4bf0_939e_a4515a84757a"  OutDataTypeStr=boolean
  Relational Operator4 : RelationalOperator  RequirementInfo="{'linktype_rmi_doors' '0000babd (/E-STEER Core/SubSystem Specifications/Application Functions/SF051A Sensor Offset Learning)' '#SF051A_125' 'true' 'REQ:  SF051A_125' '' } %GIDa_2be8b1bd_9967_4fbe_97b2_b4364b67bd3a"  Operator=<=  OutDataTypeStr=boolean
  Subsystem5 : Subsystem  Description=|  mask(Copyright Information){none=on}
      | Copyright info block.                                               
      |                                                                     
      | Place copyright information at the top of every subsystem in design.
      mask prompts: none "No parameters"
      mask help: Place copyright information at the top of every subsystem in design.
      mask Display:
      | NxtrConf = 'Nexteer Confidential';
      | 
      | sys = bdroot; %handle for the current model ("system")
      | first = get_param(sys,'Created');
      | first = first(end-3:end);  %year is last four digits
      | 
      | last = get_param(sys,'LastModifiedDate');
      | if isempty(last)
      |     last = datestr(now,'yyyy');
      | else
      |     last = last(end-3:end);
      | end
      | 
      | if strcmp(first,last)
      |     fprintf('%s -- Copyright %s Nexteer',NxtrConf,first)
      | else
      |     fprintf('%s -- %s%s- %s Nexteer',NxtrConf,char(169),first,last)
      | end
  LrngCdnVld : Outport
  wires:
  Relational Operator3/1 -> If/1
  HwVelFild/1 -> Abslt_f32_f32/1
  Relational Operator1/1 -> If/3
  Relational Operator4/1 -> If/2
  Abslt_f32_f32/1 -> Relational Operator4/1
  SysTqFild/1 -> Abslt_f32_f2/1
  Relational Operator2/1 -> If/4
  Abslt_f32_f2/1 -> Relational Operator2/1
  Abslt_f32_f1/1 -> Relational Operator1/1
  YawRateCorrd/1 -> Abslt_f32_f1/1
  Constant/1 -> Relational Operator4/2
  Constant1/1 -> Relational Operator1/2
  Constant2/1 -> Relational Operator2/2
  Constant3/1 -> Relational Operator3/2
  If/1 -> DrivingStraight/Action
  If/2 -> NotDrivingStraight/Action
  DrivingStraight/1(HwAgLrngDrvgDst) -> Merge/1
  NotDrivingStraight/1(HwAgLrngDrvgDstPrev) -> Merge/2
  Merge/1 -> Relational Operator/1, Data Store Write/1
  Calibration/1 -> Relational Operator/2
  Relational Operator/1 -> Display/1, LrngCdnVld/1
  VehSpd/1 -> DrivingStraight/1(VehSpd), Relational Operator3/1

== system SF051A_SnsrOffsLrng/SnsrOffsLrng/SnsrOffsLrngPer2/Enable_Function/POC/Reset_HwAg_Learning ==
  note: Suggest coding as inline local function: void Reset_HwAg_Learning()
  note: Set HwAg Offlset learning filter back to the last good learned value written to NVM Ram.
      | Set elapsed learning time back to zero.
  note: Reset timer
  note: Reset filters
  Action Port : ActionPort  ActionType=then
  Constant : Constant  Value=ZERO_ULS_F32  OutDataTypeStr=single
      settings: AttributesFormatString=%<OutDataTypeStr>
  Filter SV : DataStoreWrite  DataStoreName=HwAgLrngFil1  DataStoreElements=HwAgLrngFil1.FilSt
  Filter SV1 : DataStoreWrite  DataStoreName=HwAgLrngFil2  DataStoreElements=HwAgLrngFil2.FilSt
  FixdToFloat_f32_s16 : FixdToFloat/FixdToFloat_f32_s16  Param1=10
  NVMRam_Read : DataStoreRead  DataStoreName=SnsrOffsLrnd  DataStoreElements=SnsrOffsLrnd.YawRateOffs
  Read NVM Ram : DataStoreRead  DataStoreName=SnsrOffsLrnd  DataStoreElements=SnsrOffsLrnd.HwAgOffs
  Subsystem5 : Subsystem  Description=|  mask(Copyright Information){none=on}
      | Copyright info block.                                               
      |                                                                     
      | Place copyright information at the top of every subsystem in design.
      mask prompts: none "No parameters"
      mask help: Place copyright information at the top of every subsystem in design.
      mask Display:
      | NxtrConf = 'Nexteer Confidential';
      | 
      | sys = bdroot; %handle for the current model ("system")
      | first = get_param(sys,'Created');
      | first = first(end-3:end);  %year is last four digits
      | 
      | last = get_param(sys,'LastModifiedDate');
      | if isempty(last)
      |     last = datestr(now,'yyyy');
      | else
      |     last = last(end-3:end);
      | end
      | 
      | if strcmp(first,last)
      |     fprintf('%s -- Copyright %s Nexteer',NxtrConf,first)
      | else
      |     fprintf('%s -- %s%s- %s Nexteer',NxtrConf,char(169),first,last)
      | end
  Update Reference : DataStoreWrite  DataStoreName=SnsrOffsLrnd  DataStoreElements=SnsrOffsLrnd.HwAgLrngYawOffsRef
  Write NVM Ram : DataStoreWrite  DataStoreName=SnsrOffsLrnd  DataStoreElements=SnsrOffsLrnd.HwAgLrndTi
  wires:
  Constant/1 -> Write NVM Ram/1
  Read NVM Ram/1 -> FixdToFloat_f32_s16/1
  NVMRam_Read/1 -> Update Reference/1
  FixdToFloat_f32_s16/1 -> Filter SV1/1, Filter SV/1

== system SF051A_SnsrOffsLrng/SnsrOffsLrng/SnsrOffsLrngPer2/Enable_Function/POC/Subsystem5 ==

== system SF051A_SnsrOffsLrng/SnsrOffsLrng/SnsrOffsLrngPer2/Enable_Function/SOaC_HierarchyManager/POCEnabler ==
  CmnSigVld : Inport  RequirementInfo="{'linktype_rmi_doors' '0000babd (/E-STEER Core/SubSystem Specifications/Application Functions/SF051A Sensor Offset Learning)' '#SF051A_135' 'true' 'REQ:  SF051A_135' '' } %GIDa_a3a90e4b_a515_4369_8278_0f9e775efabb"
  VehYawRateVld : Inport  RequirementInfo="{'linktype_rmi_doors' '0000babd (/E-STEER Core/SubSystem Specifications/Application Functions/SF051A Sensor Offset Learning)' '#SF051A_135' 'true' 'REQ:  SF051A_135' '' } %GIDa_046d27fa_e356_4762_86a1_0902f3c2ade4"  Port=2
  YawRateOffsFrsh : Inport  RequirementInfo="{'linktype_rmi_doors' '0000babd (/E-STEER Core/SubSystem Specifications/Application Functions/SF051A Sensor Offset Learning)' '#SF051A_135' 'true' 'REQ:  SF051A_135' '' } %GIDa_03f8236f_a4d8_4504_bef2_73d121deb598"  Port=3
  Constant1 : Constant  RequirementInfo="{'linktype_rmi_doors' '0000babd (/E-STEER Core/SubSystem Specifications/Application Functions/SF051A Sensor Offset Learning)' '#SF051A_136' 'true' 'REQ:  SF051A_136' '' ; 'linktype_rmi_doors' '0000babd (/E-STEER Core/SubSystem Specifications/Application Functions/SF051A Sensor Offset Learning)' '#SF051A_135' 'true' 'REQ:  SF051A_135' '' } %GIDa_886d2d83_0f18_47ff_afe5_95719c677a16"  Value=SnsrOffsLrngHwAgLrngEna
  Display : DataStoreWrite  DataStoreName=dSnsrOffsLrngHwAgLrngEna
  Logical Operator : Logic  RequirementInfo="{'linktype_rmi_doors' '0000babd (/E-STEER Core/SubSystem Specifications/Application Functions/SF051A Sensor Offset Learning)' '#SF051A_135' 'true' 'REQ:  SF051A_135' '' ; 'linktype_rmi_doors' '0000babd (/E-STEER Core/SubSystem Specifications/Application Functions/SF051A Sensor Offset Learning)' '#SF051A_136' 'true' 'REQ:  SF051A_136' '' } %GIDa_e1d92644_86b9_417b_bb7c_d622c0b2c40b"  Inputs=5  AllPortsSameDT=off  OutDataTypeStr=boolean
  NvmRam : DataStoreRead  RequirementInfo="{'linktype_rmi_doors' '0000babd (/E-STEER Core/SubSystem Specifications/Application Functions/SF051A Sensor Offset Learning)' '#SF051A_135' 'true' 'REQ:  SF051A_135' '' } %GIDa_d64055b6_ad18_4625_99bc_bc222697d718"  DataStoreName=SnsrOffsLrnd  DataStoreElements=SnsrOffsLrnd.YawRateOffsVld
  Subsystem5 : Subsystem  Description=|  mask(Copyright Information){none=on}
      | Copyright info block.                                               
      |                                                                     
      | Place copyright information at the top of every subsystem in design.
      mask prompts: none "No parameters"
      mask help: Place copyright information at the top of every subsystem in design.
      mask Display:
      | NxtrConf = 'Nexteer Confidential';
      | 
      | sys = bdroot; %handle for the current model ("system")
      | first = get_param(sys,'Created');
      | first = first(end-3:end);  %year is last four digits
      | 
      | last = get_param(sys,'LastModifiedDate');
      | if isempty(last)
      |     last = datestr(now,'yyyy');
      | else
      |     last = last(end-3:end);
      | end
      | 
      | if strcmp(first,last)
      |     fprintf('%s -- Copyright %s Nexteer',NxtrConf,first)
      | else
      |     fprintf('%s -- %s%s- %s Nexteer',NxtrConf,char(169),first,last)
      | end
  HwAgLrngEna : Outport
  wires:
  Logical Operator/1 -> Display/1, HwAgLrngEna/1
  CmnSigVld/1 -> Logical Operator/2
  Constant1/1 -> Logical Operator/1
  YawRateOffsFrsh/1 -> Logical Operator/4
  NvmRam/1 -> Logical Operator/5
  VehYawRateVld/1 -> Logical Operator/3

== system SF051A_SnsrOffsLrng/SnsrOffsLrng/SnsrOffsLrngPer2/Enable_Function/SOaC_HierarchyManager/POCResetLogic ==
  note: Capture the learned Yaw Rate Offset each time that HwAg learning is reset.  If at any time
      | Yaw Rate Offset changes significantly from the captured reference value, reset the HwAg
      | learning routine.  In other words, a major change in Yaw triggers a re-learn of HwAg.
  Abslt_f32_f32 : NxtrAbslt/Abslt_f32_f32  RequirementInfo="{'linktype_rmi_doors' '0000babd (/E-STEER Core/SubSystem Specifications/Application Functions/SF051A Sensor Offset Learning)' '#SF051A_134' 'true' 'REQ:  SF051A_134' '' } %GIDa_eb268217_533f_429b_abe3_8ca1827af580"  SFunctionSpec=single y1 = Abslt_f32_f32(single u1)
      settings: AttributesFormatString=%<Name>
  Constant : Constant  RequirementInfo="{'linktype_rmi_doors' '0000babd (/E-STEER Core/SubSystem Specifications/Application Functions/SF051A Sensor Offset Learning)' '#SF051A_134' 'true' 'REQ:  SF051A_134' '' } %GIDa_cb9b8ced_48a1_40df_bd9e_7bf129476d0f"  Value=SnsrOffsLrngHwAgLrngYawOffsDbnd
  Data Store Read : DataStoreRead  RequirementInfo="{'linktype_rmi_doors' '0000babd (/E-STEER Core/SubSystem Specifications/Application Functions/SF051A Sensor Offset Learning)' '#SF051A_134' 'true' 'REQ:  SF051A_134' '' } %GIDa_76c40593_7955_4a5c_86c5_bdfe212e95b7"  DataStoreName=SnsrOffsLrnd  DataStoreElements=SnsrOffsLrnd.HwAgLrngYawOffsRef
  Display : DataStoreWrite  DataStoreName=dSnsrOffsLrngHwAgLrngRst
  FixdToFloat_f32_s1 : FixdToFloat/FixdToFloat_f32_s16  RequirementInfo="{'linktype_rmi_doors' '0000babd (/E-STEER Core/SubSystem Specifications/Application Functions/SF051A Sensor Offset Learning)' '#SF051A_134' 'true' 'REQ:  SF051A_134' '' } %GIDa_6455c289_ed33_4177_b6b5_a172c9b77801"  Param1=9
  FixdToFloat_f32_s16 : FixdToFloat/FixdToFloat_f32_s16  RequirementInfo="{'linktype_rmi_doors' '0000babd (/E-STEER Core/SubSystem Specifications/Application Functions/SF051A Sensor Offset Learning)' '#SF051A_134' 'true' 'REQ:  SF051A_134' '' } %GIDa_7b39a599_1da3_484b_8e4f_9eef5a9ab7b8"  Param1=9
  NVMRam_Read : DataStoreRead  RequirementInfo="{'linktype_rmi_doors' '0000babd (/E-STEER Core/SubSystem Specifications/Application Functions/SF051A Sensor Offset Learning)' '#SF051A_134' 'true' 'REQ:  SF051A_134' '' } %GIDa_7759f917_66ca_4690_a4ef_7d43ee1a0bc2"  DataStoreName=SnsrOffsLrnd  DataStoreElements=SnsrOffsLrnd.YawRateOffs
  Relational Operator : RelationalOperator  RequirementInfo="{'linktype_rmi_doors' '0000babd (/E-STEER Core/SubSystem Specifications/Application Functions/SF051A Sensor Offset Learning)' '#SF051A_134' 'true' 'REQ:  SF051A_134' '' } %GIDa_3c7dc04c_6755_4531_889f_25e567f76468"  OutDataTypeStr=boolean
  Subsystem5 : Subsystem  Description=|  mask(Copyright Information){none=on}
      | Copyright info block.                                               
      |                                                                     
      | Place copyright information at the top of every subsystem in design.
      mask prompts: none "No parameters"
      mask help: Place copyright information at the top of every subsystem in design.
      mask Display:
      | NxtrConf = 'Nexteer Confidential';
      | 
      | sys = bdroot; %handle for the current model ("system")
      | first = get_param(sys,'Created');
      | first = first(end-3:end);  %year is last four digits
      | 
      | last = get_param(sys,'LastModifiedDate');
      | if isempty(last)
      |     last = datestr(now,'yyyy');
      | else
      |     last = last(end-3:end);
      | end
      | 
      | if strcmp(first,last)
      |     fprintf('%s -- Copyright %s Nexteer',NxtrConf,first)
      | else
      |     fprintf('%s -- %s%s- %s Nexteer',NxtrConf,char(169),first,last)
      | end
  Subtract : Sum  RequirementInfo="{'linktype_rmi_doors' '0000babd (/E-STEER Core/SubSystem Specifications/Application Functions/SF051A Sensor Offset Learning)' '#SF051A_134' 'true' 'REQ:  SF051A_134' '' } %GIDa_8b9d9596_8162_48c0_9d38_f3b9f3ab54f1"  Inputs=+-
  HwAgLrngRst : Outport
  wires:
  Abslt_f32_f32/1 -> Relational Operator/1
  Subtract/1 -> Abslt_f32_f32/1
  Constant/1 -> Relational Operator/2
  NVMRam_Read/1 -> FixdToFloat_f32_s16/1
  Data Store Read/1 -> FixdToFloat_f32_s1/1
  Relational Operator/1 -> Display/1, HwAgLrngRst/1
  FixdToFloat_f32_s16/1 -> Subtract/1
  FixdToFloat_f32_s1/1 -> Subtract/2

== system SF051A_SnsrOffsLrng/SnsrOffsLrng/SnsrOffsLrngPer2/Enable_Function/SOaC_HierarchyManager/Subsystem5 ==
